simulink subsystem "Get_Frenet"  (R2022b)
settings: Solver=VariableStepAuto  StartTime=0.0  StopTime=10.0  RelTol=1e-3
settings Model: Creator=User  LastModifiedBy=User

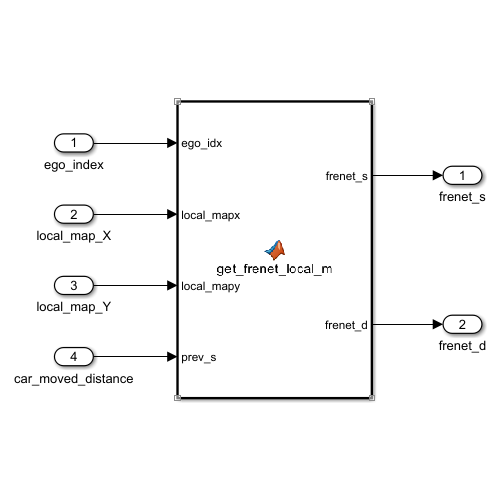
[thumbnail: Simulink's stored preview of the top-level diagram]
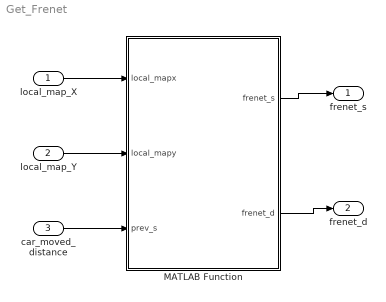
== system Get_Frenet ==
  local_map_X : Inport
  local_map_Y : Inport  Port=2
  car_moved_distance : Inport  Port=3
  MATLAB Function : MATLAB Function  TreatAsAtomicUnit=on
  frenet_s : Outport
  frenet_d : Outport  Port=2
  wires:
  local_map_X/1 -> MATLAB Function/1(local_mapx)
  local_map_Y/1 -> MATLAB Function/2(local_mapy)
  car_moved_distance/1 -> MATLAB Function/3(prev_s)
  MATLAB Function/1(frenet_s) -> frenet_s/1
  MATLAB Function/2(frenet_d) -> frenet_d/1

== matlab function Get_Frenet/MATLAB Function ==
  data: frenet_s output; local_mapx input; local_mapy input; prev_s input; frenet_d output
function [frenet_s, frenet_d] = get_frenet_local_m(local_mapx, local_mapy, prev_s)
    [frenet_s, frenet_d] = get_frenet_local(local_mapx, local_mapy, prev_s);
    
end
